simulink model "lab2_closed_loop"  (R2025b)
settings: Solver=ode45  StartTime=0.0  StopTime=400  MaxStep=0.5  RelTol=1e-3
values from neighbouring files (symbols this model uses):
  A = 14.1208    [circuit_model.m]    (also in closed_sweep.m; controller_simualtion_result.m; open_loop.m)
  K = Kvals(i)    [closed_sweep.m]    (also in controller_simualtion_result.m = 0.0122)
  ks = 0.6599    [circuit_model.m]    (also in closed_sweep.m; controller_simualtion_result.m; open_loop.m)
  r_m = 5    [circuit_model.m]    (also in closed_sweep.m; controller_simualtion_result.m)
  tau = 12.9898    [circuit_model.m]    (also in closed_sweep.m; controller_simualtion_result.m; open_loop.m)
  Vhover = 2.5    [circuit_model.m]    (also in closed_sweep.m; controller_simualtion_result.m; open_loop.m; velocity_position_plots.m)
settings Model: Creator=MTMTAD006  LastModifiedBy=MTMTAD006

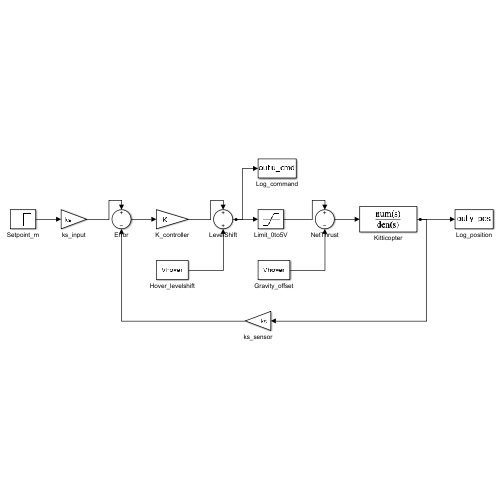
[thumbnail: Simulink's stored preview of the top-level diagram]
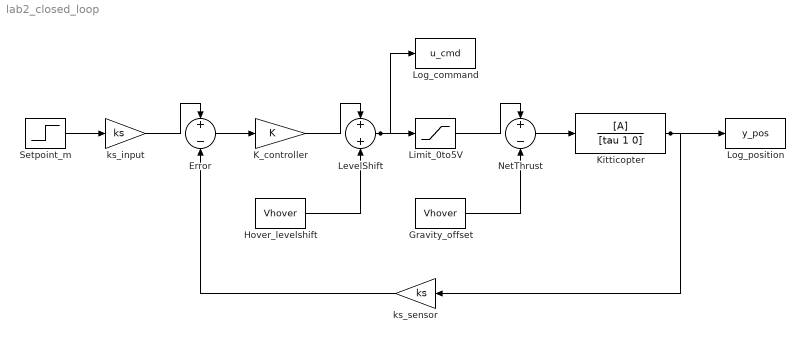
== system lab2_closed_loop ==
  Error : Sum  Inputs=+-
  Gravity_offset : Constant  Value=Vhover
  Hover_levelshift : Constant  Value=Vhover
  K_controller : Gain  Gain=K
  Kitticopter : TransferFcn  Numerator=[A]  Denominator=[tau 1 0]
  LevelShift : Sum
  Limit_0to5V : Saturate  UpperLimit=5  LowerLimit=0
  Log_command : ToWorkspace  VariableName=u_cmd  SaveFormat=Timeseries  SampleTime=-1
  Log_position : ToWorkspace  VariableName=y_pos  SaveFormat=Timeseries  SampleTime=-1
  NetThrust : Sum  Inputs=+-
  Setpoint_m : Step  Time=0  After=r_m  SampleTime=0
  ks_input : Gain  Gain=ks
  ks_sensor : Gain  Gain=ks
  wires:
  Setpoint_m/1 -> ks_input/1
  ks_input/1 -> Error/1
  Error/1 -> K_controller/1
  K_controller/1 -> LevelShift/1
  Hover_levelshift/1 -> LevelShift/2
  LevelShift/1 -> Limit_0to5V/1, Log_command/1
  Limit_0to5V/1 -> NetThrust/1
  Gravity_offset/1 -> NetThrust/2
  NetThrust/1 -> Kitticopter/1
  Kitticopter/1 -> Log_position/1, ks_sensor/1
  ks_sensor/1 -> Error/2
